simulink model "pendule_inv_capteur_etu"  (R2019a)
settings: Solver=VariableStepAuto  StartTime=0.0  StopTime=10.0  RelTol=1e-3
settings Model: Creator=tsadurni  LastModifiedBy=tsadurni

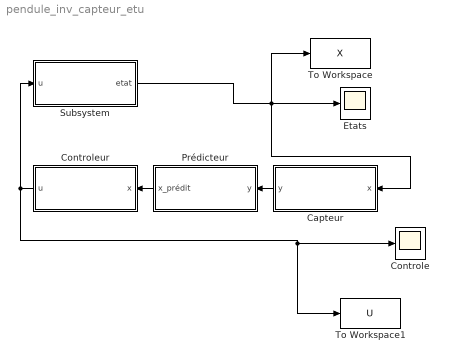
== system pendule_inv_capteur_etu ==
  Capteur : Subsystem
  "Controle " : Scope
  Controleur : Subsystem
  "Etats " : Scope
  Prédicteur : Subsystem
  Subsystem : Subsystem
  To Workspace : ToWorkspace  VariableName=X  SaveFormat=Timeseries  SampleTime=-1
  "To Workspace1 " : ToWorkspace  VariableName=U  SaveFormat=Timeseries  SampleTime=-1
  wires:
  Subsystem/1(etat) -> Capteur/1(x), To Workspace/1, "Etats "/1
  Controleur/1("u ") -> "To Workspace1 "/1, "Controle "/1, Subsystem/1(u)
  Capteur/1(y) -> Prédicteur/1("y ")
  Prédicteur/1(x_prédit) -> Controleur/1("x ")

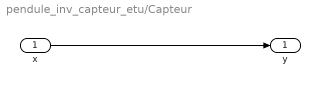
== system pendule_inv_capteur_etu/Capteur ==
  x : Inport
  y : Outport
  wires:
  x/1 -> y/1

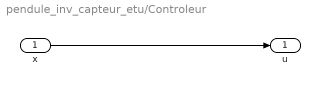
== system pendule_inv_capteur_etu/Controleur ==
  "x " : Inport
  "u " : Outport
  wires:
  "x "/1 -> "u "/1

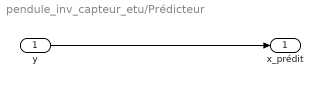
== system pendule_inv_capteur_etu/Prédicteur ==
  "y " : Inport
  x_prédit : Outport
  wires:
  "y "/1 -> x_prédit/1

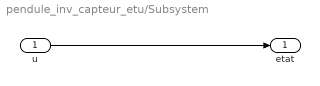
== system pendule_inv_capteur_etu/Subsystem ==
  u : Inport
  etat : Outport
  wires:
  u/1 -> etat/1
